simulink model "stateflow_test"  (R2024a)
settings: Solver=ode113  StartTime=0.0  StopTime=1500  FixedStep=1  MaxStep=1  RelTol=1e-3
libraries: simulink x1
settings Model: Creator=rzxha  LastModifiedBy=rzxha

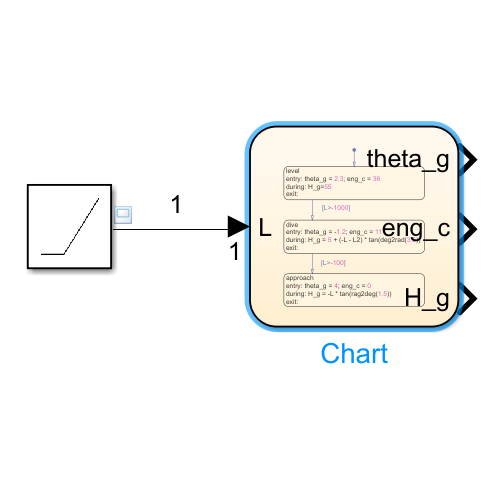
[thumbnail: Simulink's stored preview of the top-level diagram]
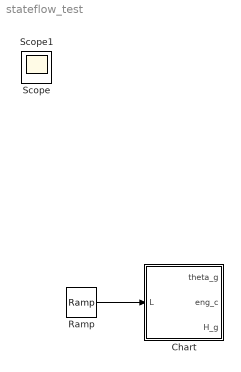
== system stateflow_test ==
  Chart : Stateflow chart  TreatAsAtomicUnit=on
  Ramp : simulink/Sources/Ramp  slope=1  start=0  InitialOutput=-1500
  Scope : Scope
  Scope1 : Scope
  wires:
  Ramp/1 -> Chart/1(L)

== stateflow chart stateflow_test/Chart ==
  state level
    entry: theta_g = 2.3; eng_c = 36
    during: H_g=55
    exit:
  state dive
    entry: theta_g = -1.2; eng_c = 11
    during: L2 = 5 / tan(deg2rad(1.5));
    H_g = 5 + (-L - L2) * tan(deg2rad(3.5))
    exit:
  state approach
    entry: theta_g = 4; eng_c = 0
    during: H_g = -L * tan(deg2rad(1.5))
    exit:
  (default) -> level
  level -> dive : [L>-1000]
  dive -> approach : [L>-100]
  data: theta_g output; eng_c output; H_g output; L input; L2 local
